simulink subsystem "GP2D12"  (R2022b)
settings: Solver=VariableStepAuto  StartTime=0.0  StopTime=10.0  RelTol=1e-3
model mask{Pin=A0}
  mask prompts: Pin "svd:svd:PinPrompt"
libraries: mbedblockslib x1
settings Model: Creator=micha  LastModifiedBy=micha

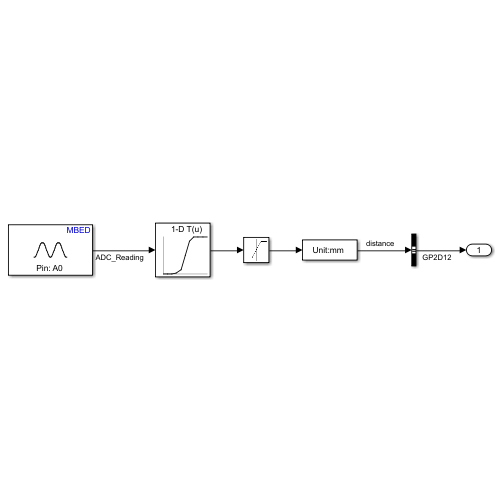
[thumbnail: Simulink's stored preview of the top-level diagram]
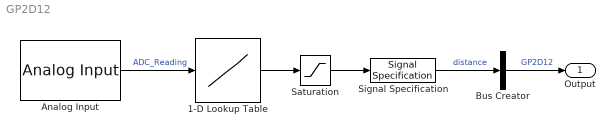
== system GP2D12 ==
  1-D Lookup Table : Lookup_n-D  NumberOfTableDimensions=1  BreakpointsForDimension1=[-5:5]  Table=tanh([-5:5])  InternalRulePriority=Speed  RndMeth=Simplest
  Analog Input : mbedblockslib/Analog Input  Pin=A1  ReadResultsOnly=off  ConversionTriggerSource=Software  ExternalTriggerType=uint32( 0 )  OutputDataType=double  EnableConversionCompleteNotify=off  EnableOuputStatus=off  SampleTime=-1
      settings: LibrarySourceBlock=stmnucleorootlib/Common/Analog Input
  Bus Creator : BusCreator  Inputs=1
  Saturation : Saturate  UpperLimit=800  LowerLimit=0
  Signal Specification : SignalSpecification  Unit=mm
  Output : Outport
  wires:
  Analog Input/1 -> 1-D Lookup Table/1  "ADC_Reading"
  1-D Lookup Table/1 -> Saturation/1
  Signal Specification/1 -> Bus Creator/1  "distance"
  Saturation/1 -> Signal Specification/1
  Bus Creator/1 -> Output/1  "GP2D12"
